simulink model "Task7"  (R2019b)
settings: Solver=VariableStepAuto  StartTime=0.0  StopTime=10.0  RelTol=1e-3
libraries: simulink x1
settings Model: Creator=12393  LastModifiedBy=12393

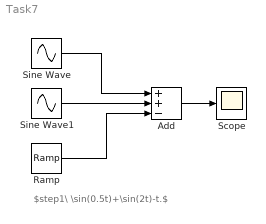
== system Task7 ==
  note: $step1\ \sin(0.5t)+\sin(2t)-t.$
  Add : Sum  Inputs=++-
  Ramp : simulink/Sources/Ramp  slope=1  start=0  InitialOutput=0
  Scope : Scope
  Sine Wave : Sin  Frequency=0.5  SampleTime=0
      settings: AttributesFormatString=Freq=%<Frequency>rad/sec
  Sine Wave1 : Sin  Frequency=2  SampleTime=0
      settings: AttributesFormatString=Freq=%<Frequency>rad/sec
  wires:
  Sine Wave/1 -> Add/1
  Sine Wave1/1 -> Add/2
  Ramp/1 -> Add/3
  Add/1 -> Scope/1
